simulink subsystem "Find_Target_Coordinate"  (R2023b)
settings: Solver=VariableStepAuto  StartTime=0.0  StopTime=10.0  RelTol=1e-3
undefined symbols (not defined in the file): Spline_Lookahead_Dist, Spline_Num_Samples
settings Model: Creator=ander  LastModifiedBy=ander

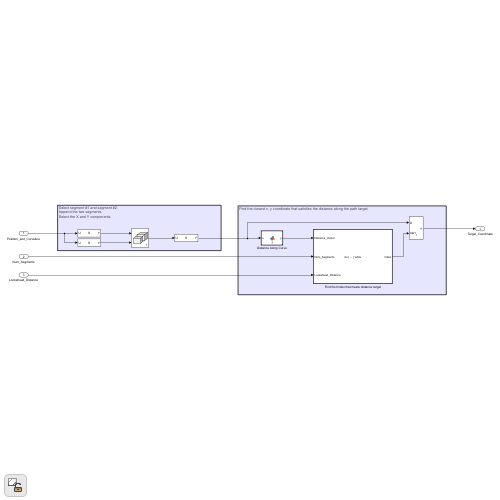
[thumbnail: Simulink's stored preview of the top-level diagram]
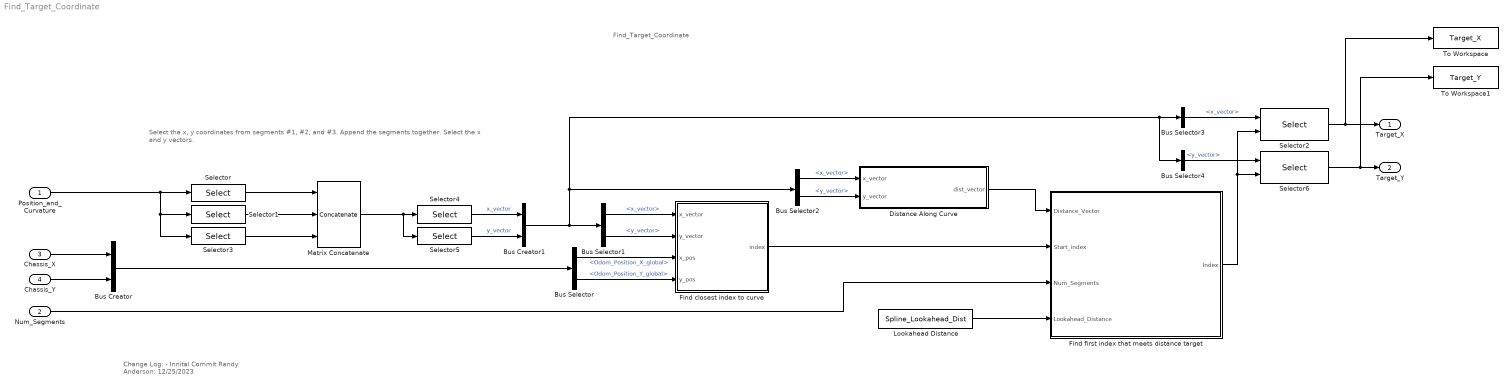
== system Find_Target_Coordinate ==
  note: Select the x, y coordinates from segments #1, #2, and #3.
      | Append the segments together.
      | Select the x and y vectors.
  note: Find_Target_Coordinate
  note: Change Log:
      | - Innital Commit
      | Randy Anderson: 12/25/2023
  Position_and_Curvature : Inport
  Num_Segments : Inport  Port=2
  Chassis_X : Inport  Port=3  OutDataTypeStr=double  Unit=m  PortDimensions=1
  Chassis_Y : Inport  Port=4  OutDataTypeStr=double  Unit=m  PortDimensions=1
  Bus Creator : BusCreator  Inputs=2
  Bus Creator1 : BusCreator  Inputs=2
  Bus Selector : BusSelector  OutputSignals=Odom_Position_X_global,Odom_Position_Y_global
  Bus Selector1 : BusSelector  OutputSignals=x_vector,y_vector
  Bus Selector2 : BusSelector  OutputSignals=x_vector,y_vector
  Bus Selector3 : BusSelector  OutputSignals=x_vector
  Bus Selector4 : BusSelector  OutputSignals=y_vector
  Distance Along Curve : MATLAB Function  TreatAsAtomicUnit=on
  Find closest index to curve : MATLAB Function  TreatAsAtomicUnit=on
  Find first index that meets distance target : Subsystem  TreatAsAtomicUnit=on
  Lookahead Distance : Constant  Value=Spline_Lookahead_Dist
  Matrix Concatenate : Concatenate  NumInputs=3  Mode=Multidimensional array
  Selector : Selector  NumberOfDimensions=3  InputPortWidth=3  IndexOptions=Select all,Index vector (dialog),Index vector (dialog)  Indices=[1 3],[1 2],1  OutputSizes=1,1,1
  Selector1 : Selector  NumberOfDimensions=3  InputPortWidth=3  IndexOptions=Select all,Index vector (dialog),Index vector (dialog)  Indices=[1 3],[1 2],2  OutputSizes=1,1,1
  Selector2 : Selector  InputPortWidth=Spline_Num_Samples_x3  IndexOptions=Index vector (port)  Indices=[1 3]  OutputSizes=1
  Selector3 : Selector  NumberOfDimensions=3  InputPortWidth=3  IndexOptions=Select all,Index vector (dialog),Index vector (dialog)  Indices=[1 3],[1 2],3  OutputSizes=1,1,1
  Selector4 : Selector  NumberOfDimensions=2  InputPortWidth=3  IndexOptions=Select all,Index vector (dialog)  Indices=[1 3],1  OutputSizes=1,1
  Selector5 : Selector  NumberOfDimensions=2  InputPortWidth=3  IndexOptions=Select all,Index vector (dialog)  Indices=[1 3],2  OutputSizes=1,1
  Selector6 : Selector  InputPortWidth=Spline_Num_Samples_x3  IndexOptions=Index vector (port)  Indices=[1 3]  OutputSizes=1
  To Workspace : ToWorkspace  VariableName=Target_X  SampleTime=-1
  To Workspace1 : ToWorkspace  VariableName=Target_Y  SampleTime=-1
  Target_X : Outport
  Target_Y : Outport  Port=2
  wires:
  Position_and_Curvature/1 -> Selector/1, Selector1/1, Selector3/1
  Selector1/1 -> Matrix Concatenate/2
  Matrix Concatenate/1 -> Selector4/1, Selector5/1
  Selector/1 -> Matrix Concatenate/1
  Distance Along Curve/1(dist_vector) -> Find first index that meets distance target/1(Distance_Vector)
  Find first index that meets distance target/1(Index) -> Selector2/2, Selector6/2
  Num_Segments/1 -> Find first index that meets distance target/3(Num_Segments)
  Selector3/1 -> Matrix Concatenate/3
  Find closest index to curve/1(index) -> Find first index that meets distance target/2(Start_index)
  Chassis_Y/1 -> Bus Creator/2
  Chassis_X/1 -> Bus Creator/1
  Bus Creator/1 -> Bus Selector/1
  Selector5/1 -> Bus Creator1/2  "y_vector"
  Selector4/1 -> Bus Creator1/1  "x_vector"
  Bus Creator1/1 -> Bus Selector1/1, Bus Selector3/1, Bus Selector4/1, Bus Selector2/1
  Bus Selector1/1 -> Find closest index to curve/1(x_vector)  "<x_vector>"
  Bus Selector1/2 -> Find closest index to curve/2(y_vector)  "<y_vector>"
  Bus Selector/2 -> Find closest index to curve/4(y_pos)  "<Odom_Position_Y_global>"
  Bus Selector/1 -> Find closest index to curve/3(x_pos)  "<Odom_Position_X_global>"
  Bus Selector2/2 -> Distance Along Curve/2(y_vector)  "<y_vector>"
  Bus Selector2/1 -> Distance Along Curve/1(x_vector)  "<x_vector>"
  Bus Selector3/1 -> Selector2/1  "<x_vector>"
  Bus Selector4/1 -> Selector6/1  "<y_vector>"
  Selector2/1 -> Target_X/1, To Workspace/1
  Selector6/1 -> Target_Y/1, To Workspace1/1
  Lookahead Distance/1 -> Find first index that meets distance target/4(Lookahead_Distance)

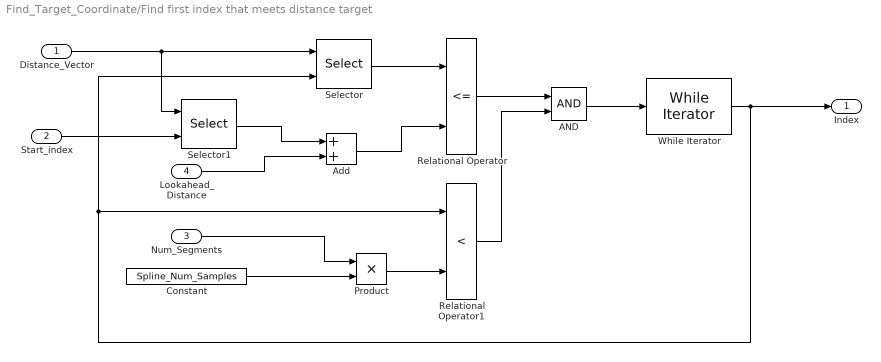
== system Find_Target_Coordinate/Find first index that meets distance target ==
  Distance_Vector : Inport
  Start_index : Inport  Port=2
  Num_Segments : Inport  Port=3
  Lookahead_Distance : Inport  Port=4
  AND : Logic  AllPortsSameDT=off  OutDataTypeStr=boolean
  Add : Sum
  Constant : Constant  Value=Spline_Num_Samples
  Product : Product
  Relational Operator : RelationalOperator  Operator=<=  OutDataTypeStr=boolean  RndMeth=Simplest  InputSameDT=off
  Relational Operator1 : RelationalOperator  Operator=<  OutDataTypeStr=boolean  RndMeth=Simplest  InputSameDT=off
  Selector : Selector  InputPortWidth=Spline_Num_Samples_x3  IndexOptions=Index vector (port)  Indices=[1 3]  OutputSizes=1
  Selector1 : Selector  InputPortWidth=Spline_Num_Samples_x3  IndexOptions=Index vector (port)  Indices=[1 3]  OutputSizes=1
  While Iterator : WhileIterator  MaxIters=Spline_Num_Samples_x3  WhileBlockType=do-while  ShowIterationPort=on  OutputDataType=uint8
  Index : Outport
  wires:
  Selector1/1 -> Add/1
  Lookahead_Distance/1 -> Add/2
  Add/1 -> Relational Operator/2
  Start_index/1 -> Selector1/2
  AND/1 -> While Iterator/1
  Relational Operator/1 -> AND/1
  Relational Operator1/1 -> AND/2
  Constant/1 -> Product/2
  Num_Segments/1 -> Product/1
  Product/1 -> Relational Operator1/2
  While Iterator/1 -> Relational Operator1/1, Selector/2, Index/1
  Selector/1 -> Relational Operator/1
  Distance_Vector/1 -> Selector/1, Selector1/1

== matlab function Find_Target_Coordinate/Distance Along Curve ==
  data: x_vector input; dist_vector output; y_vector input
function dist_vector = distance(x_vector,y_vector)
% Calculate the distance vector along the curve x, y coordinate pair
% from the first index to the last index.
%
% Randy Anderson
% 2023-12-21

len = length(x_vector);
dist_vector = zeros(len,1);
for k = 2:len
    x_delta = x_vector(k)-x_vector(k-1);
    y_delta = y_vector(k)-y_vector(k-1);
    distance = hypot(x_delta,y_delta);
    dist_vector(k) = dist_vector(k-1) + distance;
end

== matlab function Find_Target_Coordinate/Find closest index to curve ==
  data: x_vector input; index output; y_vector input; x_pos input; y_pos input
function index = find_index(x_vector,y_vector,x_pos,y_pos)
% Finds the index corresponding to input x, y vectors that is the closest
% coordinate pair along the curve to the robot x, y position.
%
% Randy Anderson
% 2023-12-23

len = length(x_vector);
distance_from_robot = zeros(len,1);
for k = 1:len
    x_delta = x_vector(k)-x_pos;
    y_delta = y_vector(k)-y_pos;
    distance_from_robot(k) = hypot(x_delta,y_delta);
end

min_distance = min(distance_from_robot);

for k = 1:len
    if distance_from_robot(k) == min_distance
        break
    end
end

index = k;
